simulink model "MCC_BO"  (R2018b)
settings: Solver=VariableStepAuto  StartTime=0.0  StopTime=0.8  MaxStep=1/(100*fn)  MinStep=1/(1000*fn)  RelTol=1e-3
values from neighbouring files (symbols this model uses):
  alfa = 3.98e-3    (= 0.00398)    [MCC_11_1_init.m]
  delta_T = 75    [MCC_11_1_init.m]
  f = Pmn/(Omega_n)^2    (= 0.114637682064)    [MCC_11_1_init.m]
  J = 6.9    [MCC_11_1_init.m]
  kc1 = 0    [MCC_11_1_init.m]
  kc2 = 0    [MCC_11_1_init.m]
  kc3 = input('Kc3 = ')    [MCC_11_1_init.m]
  L = 0.62e-3    (= 0.00062)    [MCC_11_1_init.m]
  phi_0 = (Un-R_115*In)/Omega_n    (= 6.30526411689)    [MCC_11_1_init.m]
  R0 = R_115/(1+alfa*delta_T)    (= 0.0623796688487)    [MCC_11_1_init.m]
  R_115 = 0.081    [MCC_11_1_init.m]
  to = 1    [MCC_11_1_init.m]
  Un = 600    [MCC_11_1_init.m]
  variable = 0    [MCC_11_1_init.m]
settings Model: Creator=cindyiskandar  LastModifiedBy=cindyiskandar

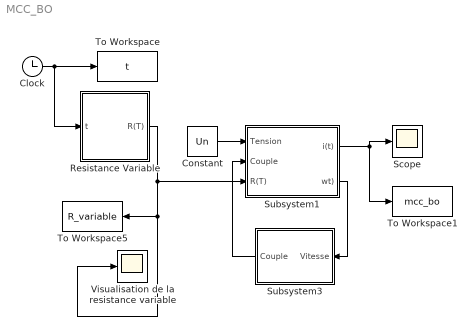
== system MCC_BO ==
  Clock : Clock
  Constant : Constant  Value=Un
  Resistance Variable : Subsystem
  Scope : Scope
  Subsystem1 : Subsystem
  Subsystem3 : Subsystem
  To Workspace : ToWorkspace  VariableName=t  SampleTime=-1
      settings: Save2DSignal=2-D array (concatenate along first dimension)
  To Workspace1 : ToWorkspace  VariableName=mcc_bo  SampleTime=-1
      settings: Save2DSignal=2-D array (concatenate along first dimension)
  To Workspace5 : ToWorkspace  VariableName=R_variable  SampleTime=-1
      settings: Save2DSignal=2-D array (concatenate along first dimension)
  Visualisation de la resistance variable : Scope
  wires:
  Subsystem1/2(wt)) -> Subsystem3/1("Vitesse ")
  Subsystem3/1("Couple ") -> Subsystem1/2(Couple)
  Subsystem1/1(i(t)) -> Scope/1, To Workspace1/1
  Constant/1 -> Subsystem1/1(Tension)
  Clock/1 -> Resistance Variable/1("t "), To Workspace/1
  Resistance Variable/1(R(T)) -> Subsystem1/3("R(T) "), To Workspace5/1, Visualisation de la resistance variable/1

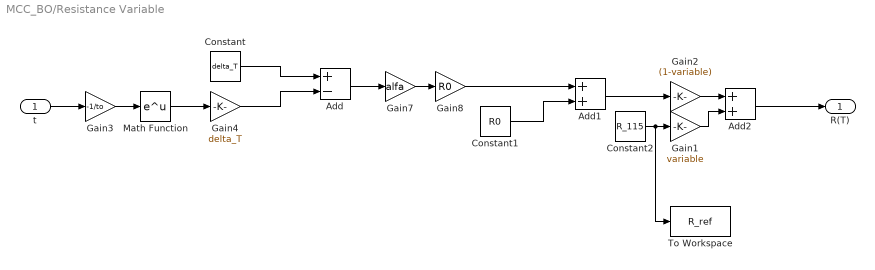
== system MCC_BO/Resistance Variable ==
  "t " : Inport
  Add : Sum  Inputs=+-
  Add1 : Sum
  Add2 : Sum
  Constant : Constant  Value=delta_T
  Constant1 : Constant  Value=R0
  Constant2 : Constant  Value=R_115
  Gain1 : Gain  Gain=variable
  Gain2 : Gain  Gain=(1-variable)
  Gain3 : Gain  Gain=-1/to
  Gain4 : Gain  Gain=delta_T
  Gain7 : Gain  Gain=alfa
  Gain8 : Gain  Gain=R0
  Math Function : Math  SaturateOnIntegerOverflow=on
  To Workspace : ToWorkspace  VariableName=R_ref  SampleTime=-1
      settings: Save2DSignal=2-D array (concatenate along first dimension)
  R(T) : Outport
  wires:
  "t "/1 -> Gain3/1
  Gain7/1 -> Gain8/1
  Add1/1 -> Gain2/1
  Gain4/1 -> Add/2
  Gain3/1 -> Math Function/1
  Gain8/1 -> Add1/1
  Constant/1 -> Add/1
  Math Function/1 -> Gain4/1
  Constant1/1 -> Add1/2
  Add/1 -> Gain7/1
  Constant2/1 -> To Workspace/1, Gain1/1
  Gain1/1 -> Add2/2
  Gain2/1 -> Add2/1
  Add2/1 -> R(T)/1

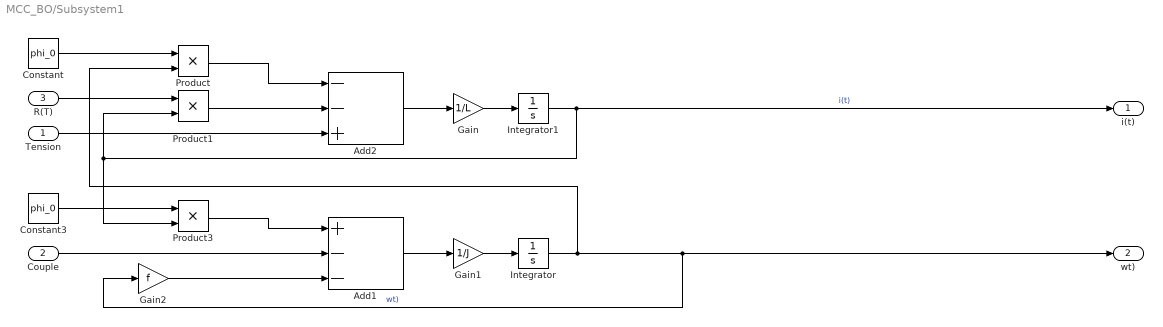
== system MCC_BO/Subsystem1 ==
  Tension : Inport
  Couple : Inport  Port=2
  "R(T) " : Inport  Port=3
  Add1 : Sum  Inputs=+--
  Add2 : Sum  Inputs=--+
  Constant : Constant  Value=phi_0
  Constant3 : Constant  Value=phi_0
  Gain : Gain  Gain=1/L
  Gain1 : Gain  Gain=1/J
  Gain2 : Gain  Gain=f
  Integrator : Integrator
  Integrator1 : Integrator
  Product : Product
  Product1 : Product
  Product3 : Product
  i(t) : Outport
  wt) : Outport  Port=2
  wires:
  Couple/1 -> Add1/2
  Gain/1 -> Integrator1/1
  Add2/1 -> Gain/1
  Product/1 -> Add2/1
  Product1/1 -> Add2/2
  "R(T) "/1 -> Product1/1
  Tension/1 -> Add2/3
  Gain1/1 -> Integrator/1
  Integrator/1 -> Gain2/1, wt)/1, Product/2  "wt)"
  Constant/1 -> Product/1
  Constant3/1 -> Product3/1
  Add1/1 -> Gain1/1
  Integrator1/1 -> i(t)/1, Product3/2, Product1/2  "i(t)"
  Product3/1 -> Add1/1
  Gain2/1 -> Add1/3

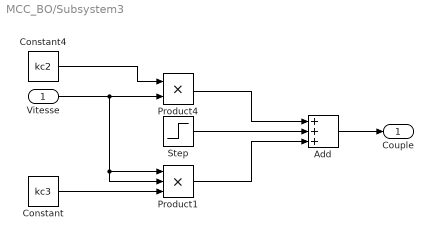
== system MCC_BO/Subsystem3 ==
  "Vitesse " : Inport
  Add : Sum  Inputs=+++
  Constant : Constant  Value=kc3
  Constant4 : Constant  Value=kc2
  Product1 : Product  Inputs=3
  Product4 : Product
  Step : Step  Time=5  After=kc1  SampleTime=0
  "Couple " : Outport
  wires:
  "Vitesse "/1 -> Product1/2, Product1/1, Product4/2
  Constant4/1 -> Product4/1
  Add/1 -> "Couple "/1
  Product4/1 -> Add/1
  Product1/1 -> Add/3
  Constant/1 -> Product1/3
  Step/1 -> Add/2
